simulink model "PMSM_R2021a"  (R2021a)
settings: Solver=FixedStepDiscrete  StartTime=0.0  StopTime=0.5  FixedStep=1e-6  MaxStep=1e-6  MinStep=1e-6  RelTol=1e-6
InitFcn:
  | Tpwm = 1e-4;%开关周期
  | Tspeed = 1e-4;%转速采样周期，在实际DSP系统中，Tspeed会小于Tpwm
  | Pn = 4;%电机极对数
  | Ls = 8.5e-3;%定子电感，采用隐极的，Ld=Lq=Ls
  | Rs = 3;%定子电阻
  | flux = 0.1688;%永磁体磁链
  | Vdc = 311;%直流母线电压
  | iqmax = 20;%额定电流
  | fc = 300;%电流环带宽
undefined symbols (not defined in the file): DiscIntNeverNeededParam
libraries: spsDCVoltageSourceLib x1, spsPermanentMagnetSynchronousMachineLib x1, simulink x1, spsUniversalBridgeLib x1, spspowerguiLib x1
settings Model: Creator=admin  LastModifiedBy=26016
settings SolverCC: AlgebraicLoopSolver=TrustRegion
settings DataIOCC: ReturnWorkspaceOutputs=off
settings DebuggingCC: ArithmeticOperatorsInVariantConditions=warning
settings SFSimCC: CustomCodeUndefinedFunction=UseInterfaceOnly
settings RTWCC: DLArmComputeVersion=20.02.1

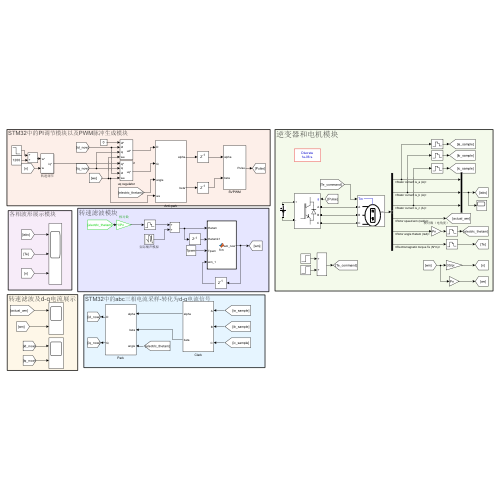
[thumbnail: Simulink's stored preview of the top-level diagram]
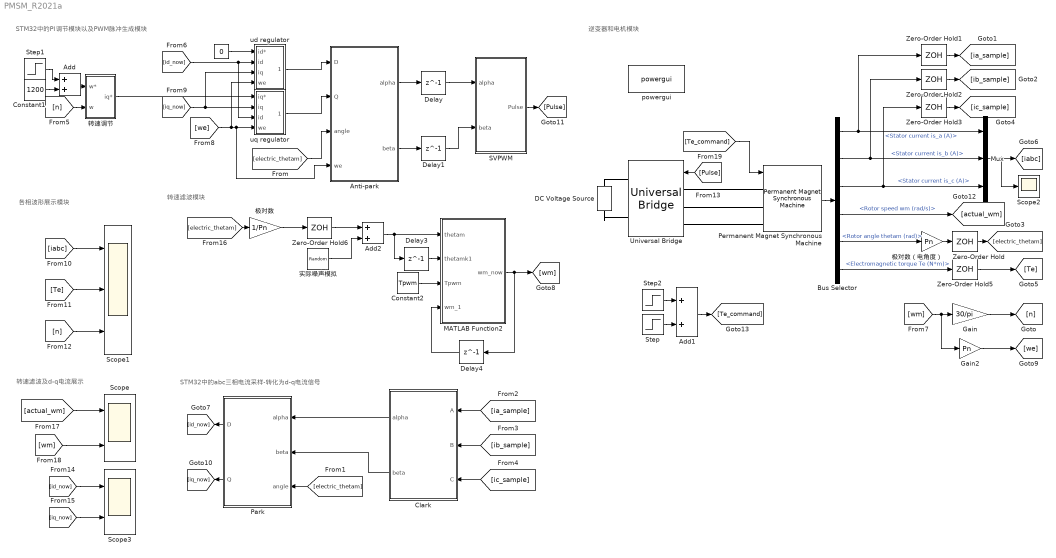
== system PMSM_R2021a ==
  note: 转速滤波模块
  note: 转速滤波及d-q电流展示
  note: 各相波形展示模块
  note: 逆变器和电机模块
  note: STM32中的PI调节模块以及PWM脉冲生成模块
  note: STM32中的abc三相电流采样-转化为d-q电流信号
  " " : Constant  Value=0
  Add : Sum
  Add1 : Sum
  Add2 : Sum
  Anti-park : Subsystem
  Bus Selector : BusSelector  OutputSignals=Stator current is_a (A),Stator current is_b (A),Stator current is_c (A),Rotor speed wm (rad/s),Rotor angle thetam (rad),Electromagnetic torque Te (N*m)
  Clark : Subsystem
  Constant1 : Constant  Value=1200
  Constant2 : Constant  Value=Tpwm
  DC Voltage Source : spsDCVoltageSourceLib/DC Voltage Source  Amplitude=Vdc  Measurements=None
  Delay{,1,3..4} (4 alike) : Delay  DelayLength=1
  Gain : Gain  Gain=30/pi
  Gain2 : Gain  Gain=Pn
  MATLAB Function2 : MATLAB Function  TreatAsAtomicUnit=on
  Mux : Mux  Inputs=3
  "Park " : Subsystem
  Permanent Magnet Synchronous Machine : spsPermanentMagnetSynchronousMachineLib/Permanent Magnet Synchronous Machine  NbPhases=3  FluxDistribution=Sinusoidal  RotorType=Round  MechanicalLoad=Torque Tm  PresetModel=No  ShowDetailedParameters=on  MeasurementBus=off  Resistance=Rs  Inductance=8.5e-3  dqInductances=[0.0009262 0.001024]  La=Ls  MachineConstant=Flux linkage established by magnets (V.s)  Flux=flux  VoltageCst=122.4677  TorqueCst=1.0128  Flat=120  Mechanical=[0.01 0.0004924 4 0]  PolePairs=4  InitialConditions=[0,0, 0,0]  InitialConditions5ph=[0 0 0 0 0 0]  RefAngle=Aligned with phase A axis (original Park)  IterativeDiscreteModel=Trapezoidal non iterative  TsBlock=-1  TsPowergui=0
  SVPWM : Subsystem
  Scope : Scope  NumInputPorts=2
  Scope1 : Scope  NumInputPorts=3
  Scope2 : Scope
  Scope3 : Scope  NumInputPorts=2
  Step : Step  Time=0.2  After=10  SampleTime=0
  Step1 : Step  Time=0.35  After=-600  SampleTime=Tpwm
  Step2 : Step  Time=0.3  After=0  SampleTime=0
  Universal Bridge : spsUniversalBridgeLib/Universal Bridge  Arms=3  SnubberResistance=1e5  SnubberCapacitance=inf  Device=IGBT / Diodes  Ron=1e-3  Lon=0  ForwardVoltages="[  0  0  ]"  ForwardVoltage=0  GTOparameters=[ 10e-6 , 20e-6 ]  IGBTparameters=[ 1e-6 , 2e-6 ]  Measurements=None  Measurements_2=None  converterType=Rectifier
  Zero-Order Hold{,1..3,5} (5 alike) : ZeroOrderHold  SampleTime=Tpwm
  Zero-Order Hold6 : ZeroOrderHold  SampleTime=Tspeed
  powergui : spspowerguiLib/powergui  Priority=1  SimulationMode=Discrete  SampleTime=1e-6  frequency=60  Iterations=50  frequencyindice=0  Pbase=100e6  ErrMax=1e-4  UnitsV=kV  UnitsW=MW  buscounter=0  FunctionMessages=off  echomessages=off  EnableUseOfTLC=off  CurrentSourceSwitches=off  DisableSnubberDevices=off  DisableRonSwitches=off  DisableVfSwitches=off  DisplayEquations=off  AutomaticDiscreteSolvers=off  SolverType=Tustin/Backward Euler (TBE)  Interpol=off  ExternalGateDelay=off  methode=off  Ts=100  x0status=blocks  SPID=off  SwTol=0  HookPort=off  NonlinearTolerance=1e-4  nMaxIteration=100  ContinueOnMaxIteration=off  RestoreLinks=warning  ResistiveCurrentMeasurement=off  Frange=[0:2:500]  Ylog=off  Xlog=on  ShowGrid=off  save=off  variable=ZData  structure=ScopeData4  ZoomFFT=on  StartTime=0.225  cycles=8  DisplayStyle=1  fundamental=80  FreqAxis=off  MaxFrequency=880  frequencyindicesteady=1  RmsSteady=1  display=off
  ud regulator : Subsystem
  "uq regulator " : Subsystem
  实际噪声模拟 : RandomNumber  Mean=0.000000025  Variance=0.000000025  SampleTime=Tpwm
  极对数 : Gain  Gain=1/Pn
  极对数（电角度） : Gain  Gain=Pn
  转速调节 : Subsystem
  wires:
  Permanent Magnet Synchronous Machine/1 -> Bus Selector/1
  Bus Selector/1 -> Mux/1, Zero-Order Hold1/1  "<Stator current is_a (A)>"
  Bus Selector/4 -> [actual_wm]  "<Rotor speed wm (rad/s)>"
  Bus Selector/2 -> Mux/2, Zero-Order Hold2/1  "<Stator current is_b (A)>"
  Bus Selector/3 -> Mux/3, Zero-Order Hold3/1  "<Stator current is_c (A)>"
  Bus Selector/6 -> Zero-Order Hold5/1  "<Electromagnetic torque Te (N*m)>"
  ud regulator/1("ud* ") -> Anti-park/1(D)
  " "/1 -> ud regulator/1(id*)
  Anti-park/1(alpha) -> Delay/1
  Anti-park/2(beta) -> Delay1/1
  Clark/1(alpha) -> "Park "/1(alpha)
  Clark/2(beta) -> "Park "/2(beta)
  "uq regulator "/1("uq* ") -> Anti-park/2(Q)
  转速调节/1("iq* ") -> "uq regulator "/1(iq*)
  极对数（电角度）/1 -> Zero-Order Hold/1
  Zero-Order Hold/1 -> [electric_thetam]
  [electric_thetam] -> Anti-park/3(angle)
  [electric_thetam] -> "Park "/3(angle)
  Zero-Order Hold1/1 -> [ia_sample]
  Zero-Order Hold2/1 -> [ib_sample]
  Zero-Order Hold3/1 -> [ic_sample]
  [ia_sample] -> Clark/1(A)
  [ib_sample] -> Clark/2(B)
  [ic_sample] -> Clark/3(C)
  Zero-Order Hold5/1 -> [Te]
  [n] -> 转速调节/2(w)
  Mux/1 -> Scope2/1, [iabc]
  "Park "/1(D) -> [id_now]
  [id_now] -> "uq regulator "/3(id), ud regulator/2(id)
  Gain/1 -> [n]
  [wm] -> Gain2/1, Gain/1
  Gain2/1 -> [we]
  [we] -> ud regulator/4(we), Anti-park/4(we), "uq regulator "/4(we)
  "Park "/2(Q) -> [iq_now]
  [iq_now] -> ud regulator/3(iq), "uq regulator "/2("iq ")
  [iabc] -> Scope1/1
  [Te] -> Scope1/2
  [n] -> Scope1/3
  Delay/1 -> SVPWM/1(alpha)
  Delay1/1 -> SVPWM/2(beta)
  SVPWM/1(Pulse) -> [Pulse]
  [Pulse] -> Universal Bridge/1
  Add/1 -> 转速调节/1(w*)
  Constant1/1 -> Add/2
  [id_now] -> Scope3/1
  [iq_now] -> Scope3/2
  Bus Selector/5 -> 极对数（电角度）/1  "<Rotor angle thetam (rad)>"
  Step1/1 -> Add/1
  极对数/1 -> Zero-Order Hold6/1
  实际噪声模拟/1 -> Add2/2
  Zero-Order Hold6/1 -> Add2/1
  [electric_thetam] -> 极对数/1
  Add2/1 -> Delay3/1, MATLAB Function2/1(thetam)
  Delay3/1 -> MATLAB Function2/2(thetamk1)
  Constant2/1 -> MATLAB Function2/3(Tpwm)
  MATLAB Function2/1(wm_now) -> Delay4/1, [wm]
  Delay4/1 -> MATLAB Function2/4(wm_1)
  [actual_wm] -> Scope/1
  [wm] -> Scope/2
  Step/1 -> Add1/2
  Step2/1 -> Add1/1
  Add1/1 -> [Te_command]
  [Te_command] -> Permanent Magnet Synchronous Machine/1
  connections:
  Universal Bridge/RConn1 -- DC Voltage Source/RConn1
  DC Voltage Source/LConn1 -- Universal Bridge/RConn2
  Permanent Magnet Synchronous Machine/LConn1 -- Universal Bridge/LConn1
  Permanent Magnet Synchronous Machine/LConn2 -- Universal Bridge/LConn2
  Permanent Magnet Synchronous Machine/LConn3 -- Universal Bridge/LConn3

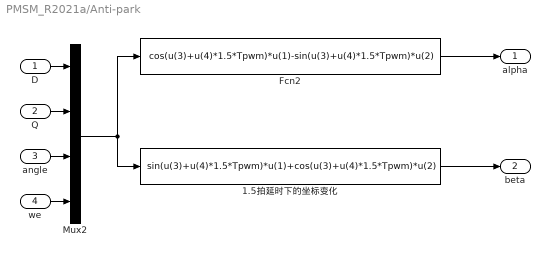
== system PMSM_R2021a/Anti-park ==
  D : Inport
  Q : Inport  Port=2
  angle : Inport  Port=3
  we : Inport  Port=4
  1.5拍延时下的坐标变化 : Fcn  Expr=sin(u(3)+u(4)*1.5*Tpwm)*u(1)+cos(u(3)+u(4)*1.5*Tpwm)*u(2)
  Fcn2 : Fcn  Expr=cos(u(3)+u(4)*1.5*Tpwm)*u(1)-sin(u(3)+u(4)*1.5*Tpwm)*u(2)
  Mux2 : Mux
  alpha : Outport  VectorParamsAs1DForOutWhenUnconnected=off
  beta : Outport  Port=2  VectorParamsAs1DForOutWhenUnconnected=off
  wires:
  angle/1 -> Mux2/3
  Mux2/1 -> Fcn2/1, 1.5拍延时下的坐标变化/1
  Fcn2/1 -> alpha/1
  1.5拍延时下的坐标变化/1 -> beta/1
  D/1 -> Mux2/1
  Q/1 -> Mux2/2
  we/1 -> Mux2/4

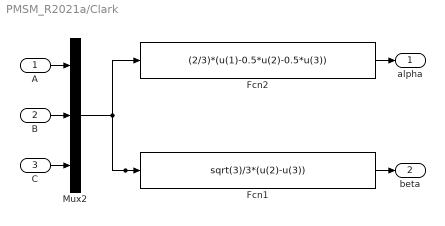
== system PMSM_R2021a/Clark ==
  A : Inport
  B : Inport  Port=2
  C : Inport  Port=3
  Fcn1 : Fcn  Expr=sqrt(3)/3*(u(2)-u(3))
  Fcn2 : Fcn  Expr=(2/3)*(u(1)-0.5*u(2)-0.5*u(3))
  Mux2 : Mux  Inputs=3
  alpha : Outport  VectorParamsAs1DForOutWhenUnconnected=off
  beta : Outport  Port=2  VectorParamsAs1DForOutWhenUnconnected=off
  wires:
  C/1 -> Mux2/3
  Fcn2/1 -> alpha/1
  Fcn1/1 -> beta/1
  A/1 -> Mux2/1
  B/1 -> Mux2/2
  Mux2/1 -> Fcn1/1, Fcn2/1

== system PMSM_R2021a/Park  ==
  alpha : Inport
  beta : Inport  Port=2
  angle : Inport  Port=3
  Fcn1 : Fcn  Expr=-sin(u(3))*u(1)+cos(u(3))*u(2)
  Fcn2 : Fcn  Expr=cos(u(3))*u(1)+sin(u(3))*u(2)
  Mux2 : Mux  Inputs=3
  D : Outport  VectorParamsAs1DForOutWhenUnconnected=off
  Q : Outport  Port=2  VectorParamsAs1DForOutWhenUnconnected=off
  wires:
  angle/1 -> Mux2/3
  Mux2/1 -> Fcn2/1, Fcn1/1
  Fcn2/1 -> D/1
  Fcn1/1 -> Q/1
  alpha/1 -> Mux2/1
  beta/1 -> Mux2/2

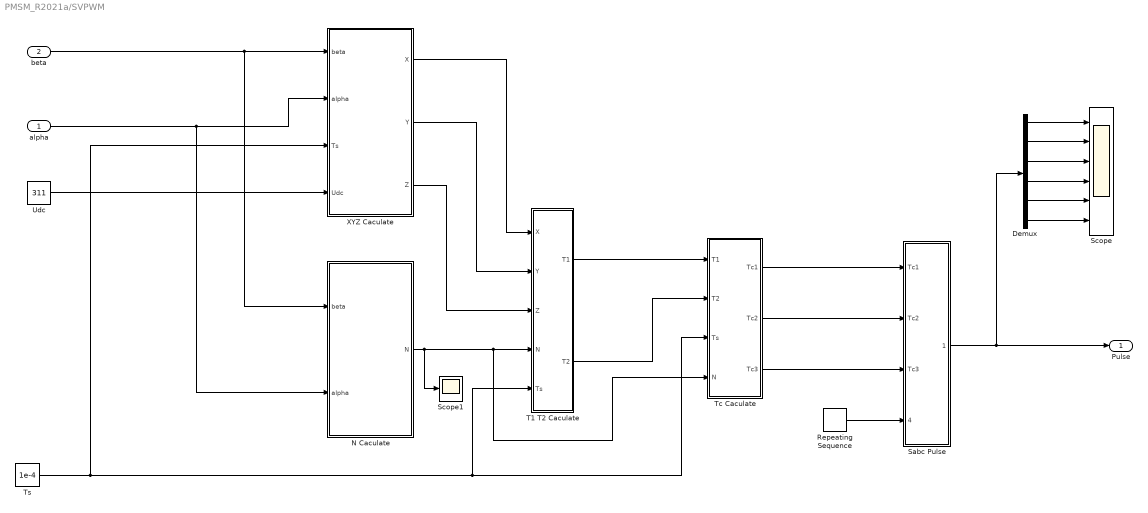
== system PMSM_R2021a/SVPWM ==
  alpha : Inport
  beta : Inport  Port=2
  Demux : Demux  Outputs=6
  N Caculate : Subsystem
  Repeating Sequence : simulink/Sources/Repeating Sequence  rep_seq_t=[0 0.00005 0.0001]  rep_seq_y=[0 0.00005 0]
  Sabc Pulse : Subsystem
  Scope : Scope  NumInputPorts=6
  Scope1 : Scope
  T1 T2 Caculate : Subsystem
  Tc Caculate : Subsystem
  Ts : Constant  Value=1e-4
  "Udc " : Constant  Value=311
  XYZ Caculate : Subsystem
  Pulse : Outport  VectorParamsAs1DForOutWhenUnconnected=off
  wires:
  beta/1 -> N Caculate/1(beta), XYZ Caculate/1(beta)
  alpha/1 -> N Caculate/2(alpha), XYZ Caculate/2(alpha)
  XYZ Caculate/1(X) -> T1 T2 Caculate/1(X)
  XYZ Caculate/2(Y) -> T1 T2 Caculate/2(Y)
  XYZ Caculate/3(Z) -> T1 T2 Caculate/3(Z)
  N Caculate/1(N) -> Scope1/1, Tc Caculate/4(N), T1 T2 Caculate/4(N)
  Ts/1 -> XYZ Caculate/3("Ts "), Tc Caculate/3(Ts), T1 T2 Caculate/5("Ts ")
  T1 T2 Caculate/1(T1) -> Tc Caculate/1(T1)
  T1 T2 Caculate/2(T2) -> Tc Caculate/2(T2)
  Tc Caculate/1(Tc1) -> Sabc Pulse/1(Tc1)
  Tc Caculate/2(Tc2) -> Sabc Pulse/2(Tc2)
  Tc Caculate/3(Tc3) -> Sabc Pulse/3(Tc3)
  Sabc Pulse/1("Pulse ") -> Demux/1, Pulse/1
  "Udc "/1 -> XYZ Caculate/4(Udc)
  Repeating Sequence/1 -> Sabc Pulse/4(Wave)
  Demux/1 -> Scope/1
  Demux/2 -> Scope/2
  Demux/3 -> Scope/3
  Demux/4 -> Scope/4
  Demux/5 -> Scope/5
  Demux/6 -> Scope/6

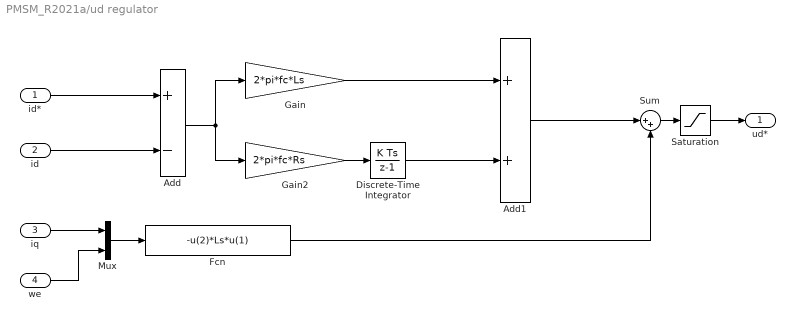
== system PMSM_R2021a/ud regulator ==
  id* : Inport
  id : Inport  Port=2
  iq : Inport  Port=3
  we : Inport  Port=4
  Add : Sum  Inputs=+-
  Add1 : Sum
  Discrete-Time Integrator : DiscreteIntegrator  SampleTime=Tpwm  LimitOutput=on  UpperSaturationLimit=Vdc/sqrt(3)  LowerSaturationLimit=-Vdc/sqrt(3)  ICPrevOutput=DiscIntNeverNeededParam  ICPrevScaledInput=DiscIntNeverNeededParam
  Fcn : Fcn  Expr=-u(2)*Ls*u(1)
  Gain : Gain  Gain=2*pi*fc*Ls
  Gain2 : Gain  Gain=2*pi*fc*Rs
  Mux : Mux  Inputs=2
  Saturation : Saturate  UpperLimit=Vdc/sqrt(3)  LowerLimit=-Vdc/sqrt(3)
  Sum : Sum  Inputs=|++
  "ud* " : Outport  VectorParamsAs1DForOutWhenUnconnected=off
  wires:
  we/1 -> Mux/2
  iq/1 -> Mux/1
  id*/1 -> Add/1
  id/1 -> Add/2
  Mux/1 -> Fcn/1
  Add1/1 -> Sum/1
  Fcn/1 -> Sum/2
  Sum/1 -> Saturation/1
  Saturation/1 -> "ud* "/1
  Gain/1 -> Add1/1
  Gain2/1 -> Discrete-Time Integrator/1
  Discrete-Time Integrator/1 -> Add1/2
  Add/1 -> Gain2/1, Gain/1

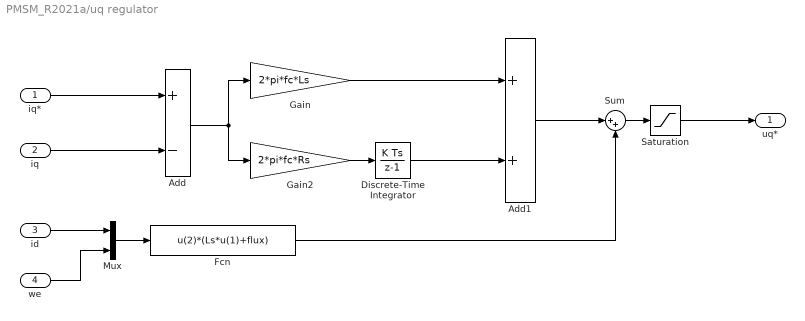
== system PMSM_R2021a/uq regulator  ==
  iq* : Inport
  "iq " : Inport  Port=2
  id : Inport  Port=3
  we : Inport  Port=4
  Add : Sum  Inputs=+-
  Add1 : Sum
  Discrete-Time Integrator : DiscreteIntegrator  SampleTime=Tpwm  LimitOutput=on  UpperSaturationLimit=Vdc/sqrt(3)  LowerSaturationLimit=-Vdc/sqrt(3)  ICPrevOutput=DiscIntNeverNeededParam  ICPrevScaledInput=DiscIntNeverNeededParam
  Fcn : Fcn  Expr=u(2)*(Ls*u(1)+flux)
  Gain : Gain  Gain=2*pi*fc*Ls
  Gain2 : Gain  Gain=2*pi*fc*Rs
  Mux : Mux  Inputs=2
  Saturation : Saturate  UpperLimit=Vdc/sqrt(3)  LowerLimit=-Vdc/sqrt(3)  LinearizeAsGain=off
  Sum : Sum  Inputs=|++
  "uq* " : Outport  VectorParamsAs1DForOutWhenUnconnected=off
  wires:
  id/1 -> Mux/1
  we/1 -> Mux/2
  "iq "/1 -> Add/2
  iq*/1 -> Add/1
  Mux/1 -> Fcn/1
  Add/1 -> Gain/1, Gain2/1
  Add1/1 -> Sum/1
  Gain2/1 -> Discrete-Time Integrator/1
  Discrete-Time Integrator/1 -> Add1/2
  Gain/1 -> Add1/1
  Fcn/1 -> Sum/2
  Sum/1 -> Saturation/1
  Saturation/1 -> "uq* "/1

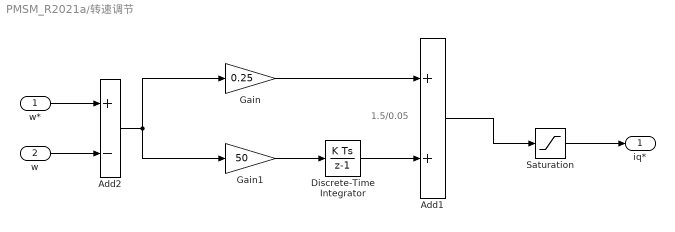
== system PMSM_R2021a/转速调节 ==
  note: 1.5/0.05
  w* : Inport
  w : Inport  Port=2
  Add1 : Sum
  Add2 : Sum  Inputs=+-
  Discrete-Time Integrator : DiscreteIntegrator  SampleTime=Tspeed  LimitOutput=on  UpperSaturationLimit=iqmax  LowerSaturationLimit=-iqmax  ICPrevOutput=DiscIntNeverNeededParam  ICPrevScaledInput=DiscIntNeverNeededParam
  Gain : Gain  Gain=0.25
  Gain1 : Gain  Gain=50
  Saturation : Saturate  UpperLimit=iqmax  LowerLimit=-iqmax
  "iq* " : Outport  VectorParamsAs1DForOutWhenUnconnected=off
  wires:
  w*/1 -> Add2/1
  Add1/1 -> Saturation/1
  Saturation/1 -> "iq* "/1
  Discrete-Time Integrator/1 -> Add1/2
  Gain/1 -> Add1/1
  w/1 -> Add2/2
  Gain1/1 -> Discrete-Time Integrator/1
  Add2/1 -> Gain1/1, Gain/1

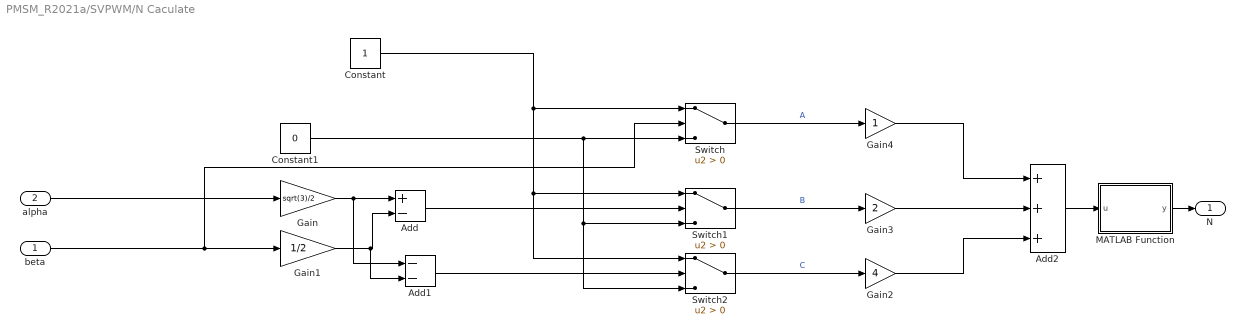
== system PMSM_R2021a/SVPWM/N Caculate ==
  beta : Inport
  alpha : Inport  Port=2
  Add : Sum  Inputs=+-
  Add1 : Sum  Inputs=--
  Add2 : Sum  Inputs=+++
  Constant : Constant
  Constant1 : Constant  Value=0
  Gain : Gain  Gain=sqrt(3)/2
  Gain1 : Gain  Gain=1/2
  Gain2 : Gain  Gain=4
  Gain3 : Gain  Gain=2
  Gain4 : Gain
  MATLAB Function : MATLAB Function  TreatAsAtomicUnit=on
  Switch : Switch  Criteria=u2 > Threshold
  Switch1 : Switch  Criteria=u2 > Threshold
  Switch2 : Switch  Criteria=u2 > Threshold
  N : Outport  VectorParamsAs1DForOutWhenUnconnected=off
  wires:
  Switch/1 -> Gain4/1  "A"
  Add/1 -> Switch1/2
  Gain/1 -> Add1/1, Add/1
  Gain3/1 -> Add2/2
  Gain2/1 -> Add2/3
  Constant/1 -> Switch/1, Switch2/1, Switch1/1
  Add1/1 -> Switch2/2
  Gain1/1 -> Add1/2, Add/2
  Add2/1 -> MATLAB Function/1(u)
  Constant1/1 -> Switch2/3, Switch1/3, Switch/3
  Gain4/1 -> Add2/1
  beta/1 -> Switch/2, Gain1/1
  Switch2/1 -> Gain2/1  "C"
  Switch1/1 -> Gain3/1  "B"
  alpha/1 -> Gain/1
  MATLAB Function/1(y) -> N/1

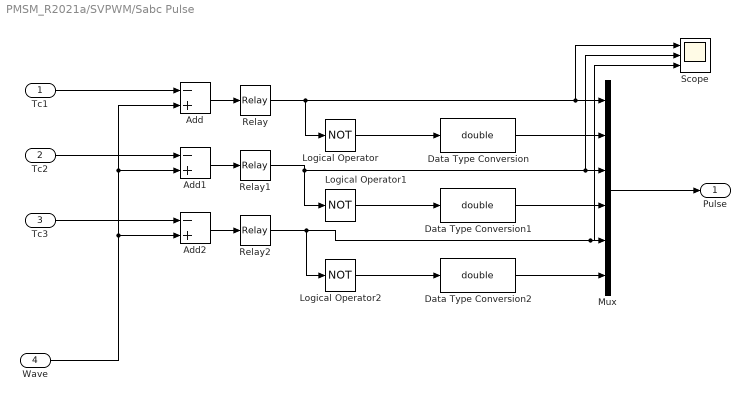
== system PMSM_R2021a/SVPWM/Sabc Pulse ==
  Tc1 : Inport
  Tc2 : Inport  Port=2
  Tc3 : Inport  Port=3
  Wave : Inport  Port=4
  Add : Sum  Inputs=-+
  Add1 : Sum  Inputs=-+
  Add2 : Sum  Inputs=-+
  Data Type Conversion : DataTypeConversion  OutDataTypeStr=double
  Data Type Conversion1 : DataTypeConversion  OutDataTypeStr=double
  Data Type Conversion2 : DataTypeConversion  OutDataTypeStr=double
  Logical Operator : Logic  Operator=NOT  AllPortsSameDT=off  OutDataTypeStr=boolean
  Logical Operator1 : Logic  Operator=NOT  AllPortsSameDT=off  OutDataTypeStr=boolean
  Logical Operator2 : Logic  Operator=NOT  AllPortsSameDT=off  OutDataTypeStr=boolean
  Mux : Mux  Inputs=6
  Relay : Relay
  Relay1 : Relay
  Relay2 : Relay
  Scope : Scope  NumInputPorts=3
  "Pulse " : Outport  VectorParamsAs1DForOutWhenUnconnected=off
  wires:
  Add/1 -> Relay/1
  Add1/1 -> Relay1/1
  Wave/1 -> Add2/2, Add1/2, Add/2
  Tc2/1 -> Add1/1
  Tc1/1 -> Add/1
  Tc3/1 -> Add2/1
  Logical Operator/1 -> Data Type Conversion/1
  Logical Operator1/1 -> Data Type Conversion1/1
  Add2/1 -> Relay2/1
  Logical Operator2/1 -> Data Type Conversion2/1
  Mux/1 -> "Pulse "/1
  Relay/1 -> Scope/1, Mux/1, Logical Operator/1
  Relay1/1 -> Scope/2, Mux/3, Logical Operator1/1
  Relay2/1 -> Logical Operator2/1, Scope/3, Mux/5
  Data Type Conversion/1 -> Mux/2
  Data Type Conversion1/1 -> Mux/4
  Data Type Conversion2/1 -> Mux/6

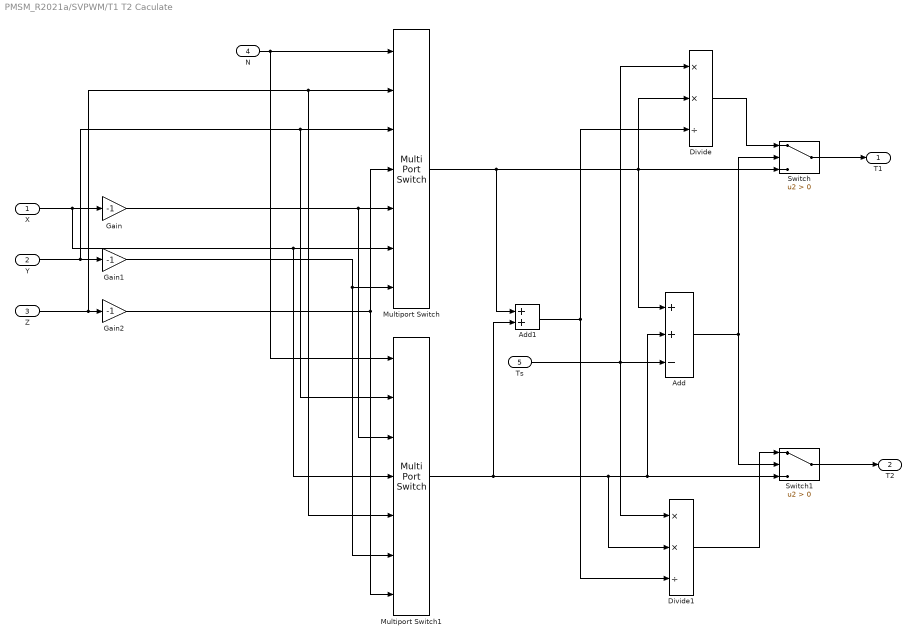
== system PMSM_R2021a/SVPWM/T1 T2 Caculate ==
  X : Inport
  Y : Inport  Port=2
  Z : Inport  Port=3
  N : Inport  Port=4
  "Ts " : Inport  Port=5
  Add : Sum  Inputs=++-
  Add1 : Sum
  Divide : Product  Inputs=**/
  Divide1 : Product  Inputs=**/
  Gain : Gain  Gain=-1
  Gain1 : Gain  Gain=-1
  Gain2 : Gain  Gain=-1
  Multiport Switch : MultiPortSwitch  Inputs=6
  Multiport Switch1 : MultiPortSwitch  Inputs=6
  Switch : Switch  Criteria=u2 > Threshold
  Switch1 : Switch  Criteria=u2 > Threshold
  T1 : Outport  VectorParamsAs1DForOutWhenUnconnected=off
  T2 : Outport  Port=2  VectorParamsAs1DForOutWhenUnconnected=off
  wires:
  Y/1 -> Multiport Switch1/2, Multiport Switch/3, Gain1/1
  X/1 -> Multiport Switch1/4, Multiport Switch/6, Gain/1
  N/1 -> Multiport Switch/1, Multiport Switch1/1
  Z/1 -> Multiport Switch1/5, Multiport Switch/2, Gain2/1
  Gain2/1 -> Multiport Switch1/7, Multiport Switch/4
  Gain/1 -> Multiport Switch1/3, Multiport Switch/5
  Gain1/1 -> Multiport Switch1/6, Multiport Switch/7
  Multiport Switch/1 -> Add1/1, Divide/2, Add/1, Switch/3
  Multiport Switch1/1 -> Add1/2, Divide1/2, Add/2, Switch1/3
  "Ts "/1 -> Divide1/1, Divide/1, Add/3
  Add/1 -> Switch1/2, Switch/2
  Divide/1 -> Switch/1
  Add1/1 -> Divide/3, Divide1/3
  Switch/1 -> T1/1
  Switch1/1 -> T2/1
  Divide1/1 -> Switch1/1

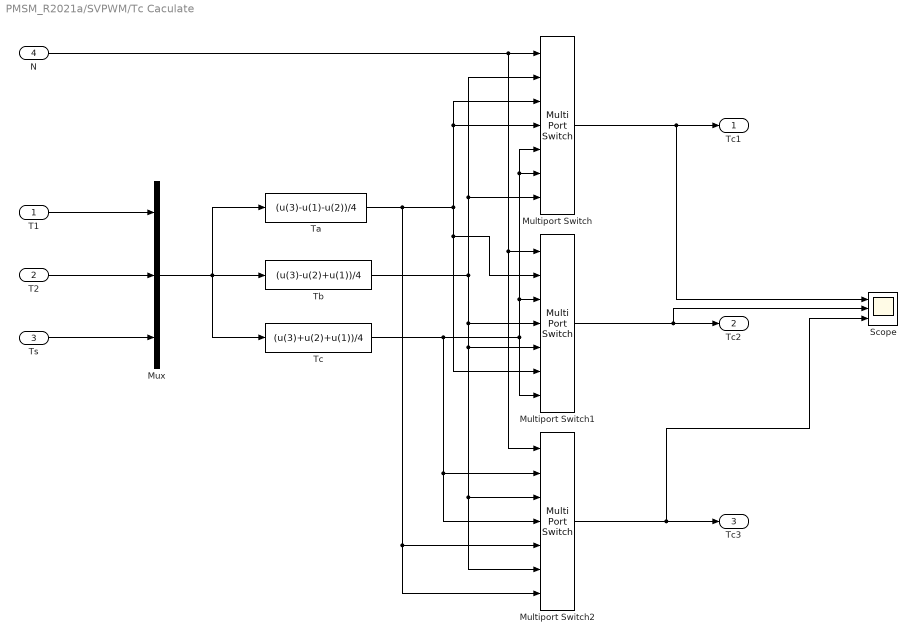
== system PMSM_R2021a/SVPWM/Tc Caculate ==
  T1 : Inport
  T2 : Inport  Port=2
  Ts : Inport  Port=3
  N : Inport  Port=4
  Multiport Switch : MultiPortSwitch  Inputs=6
  Multiport Switch1 : MultiPortSwitch  Inputs=6
  Multiport Switch2 : MultiPortSwitch  Inputs=6
  Mux : Mux  Inputs=3
  Scope : Scope  NumInputPorts=3
  Ta : Fcn  Expr=(u(3)-u(1)-u(2))/4
  Tb : Fcn  Expr=(u(3)-u(2)+u(1))/4
  Tc : Fcn  Expr=(u(3)+u(2)+u(1))/4
  Tc1 : Outport  VectorParamsAs1DForOutWhenUnconnected=off
  Tc2 : Outport  Port=2  VectorParamsAs1DForOutWhenUnconnected=off
  Tc3 : Outport  Port=3  VectorParamsAs1DForOutWhenUnconnected=off
  wires:
  T2/1 -> Mux/2
  T1/1 -> Mux/1
  Ts/1 -> Mux/3
  Mux/1 -> Tc/1, Ta/1, Tb/1
  N/1 -> Multiport Switch2/1, Multiport Switch1/1, Multiport Switch/1
  Ta/1 -> Multiport Switch2/7, Multiport Switch2/5, Multiport Switch/3, Multiport Switch/4, Multiport Switch1/6, Multiport Switch1/2
  Tb/1 -> Multiport Switch/7, Multiport Switch/2, Multiport Switch1/4, Multiport Switch2/6, Multiport Switch2/3, Multiport Switch1/5
  Tc/1 -> Multiport Switch2/4, Multiport Switch2/2, Multiport Switch1/7, Multiport Switch1/3, Multiport Switch/6, Multiport Switch/5
  Multiport Switch/1 -> Scope/1, Tc1/1
  Multiport Switch1/1 -> Scope/2, Tc2/1
  Multiport Switch2/1 -> Scope/3, Tc3/1

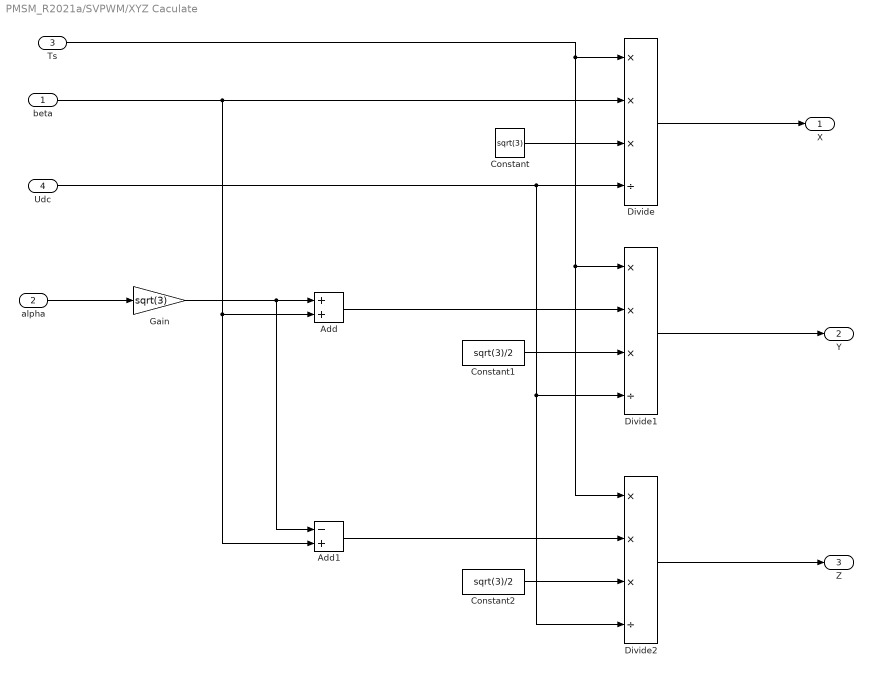
== system PMSM_R2021a/SVPWM/XYZ Caculate ==
  beta : Inport
  alpha : Inport  Port=2
  "Ts " : Inport  Port=3
  Udc : Inport  Port=4
  Add : Sum
  Add1 : Sum  Inputs=-+
  Constant : Constant  Value=sqrt(3)
  Constant1 : Constant  Value=sqrt(3)/2
  Constant2 : Constant  Value=sqrt(3)/2
  Divide : Product  Inputs=***/
  Divide1 : Product  Inputs=***/
  Divide2 : Product  Inputs=***/
  Gain : Gain  Gain=sqrt(3)
  X : Outport  VectorParamsAs1DForOutWhenUnconnected=off
  Y : Outport  Port=2  VectorParamsAs1DForOutWhenUnconnected=off
  Z : Outport  Port=3  VectorParamsAs1DForOutWhenUnconnected=off
  wires:
  "Ts "/1 -> Divide2/1, Divide1/1, Divide/1
  Udc/1 -> Divide1/4, Divide2/4, Divide/4
  Constant/1 -> Divide/3
  beta/1 -> Add1/2, Add/2, Divide/2
  Constant2/1 -> Divide2/3
  Constant1/1 -> Divide1/3
  Add/1 -> Divide1/2
  Add1/1 -> Divide2/2
  Gain/1 -> Add1/1, Add/1
  alpha/1 -> Gain/1
  Divide1/1 -> Y/1
  Divide/1 -> X/1
  Divide2/1 -> Z/1

== matlab function PMSM_R2021a/SVPWM/N Caculate/MATLAB Function ==
  data: u input; y output
function y = fcn(u)
if u==0
    y=1;
else
    y = u;
end

== matlab function PMSM_R2021a/MATLAB Function2 ==
  data: thetam input; wm_now output; thetamk1 input; Tpwm input; wm_1 input
function wm_now = fcn(thetam,thetamk1,Tpwm,wm_1)

wm = (thetam-thetamk1)/Tpwm;

%离散化低通滤波器的参考网站：
%https://www.zhihu.com/search?type=content&q=%E7%A6%BB%E6%95%A3%E5%8C%96%E4%BD%8E%E9%80%9A%E6%BB%A4%E6%B3%A2%E5%99%A8
%根据论文中选择低通滤波器截止频率为150Hz，所以可以计算出下列的低通滤波系数
low_pass_factor1 = 2*pi*150*Tpwm;
low_pass_factor2 = low_pass_factor1/(1+low_pass_factor1);

%离散化的低通滤波器的表达式
wm_now = low_pass_factor2*wm+(1-low_pass_factor2)*wm_1;


end
